simulink model "REALTIME_PART1_backwardEuler"  (R2020b)
settings: Solver=ode3  StartTime=0.0  StopTime=5  FixedStep=0.001  RelTol=1e-3
undefined symbols (not defined in the file or in its folder): ctrl, DiscIntNeverNeededParam, K_w, National_Instruments, PCI, sens, step_size, T, Tl
libraries: sldrtlib x2
settings Model: ExtModeTrigDuration=6000  Creator=gioel  LastModifiedBy=pavarinlau
settings DataIOCC: ReturnWorkspaceOutputs=off
settings RTWCC: Description=Simulink Desktop Real-Time  SystemTargetFile=sldrt.tlc  TemplateMakefile=sldrt.tmf  RTWCompilerOptimization=on
settings CodeAppCC: MaxIdLength=95
settings SimulinkDesktopRealTimeCC: TargetPreCompLibLocation=C:\Program Files\MATLAB\R2020b\toolbox\sldrt\lib\win64

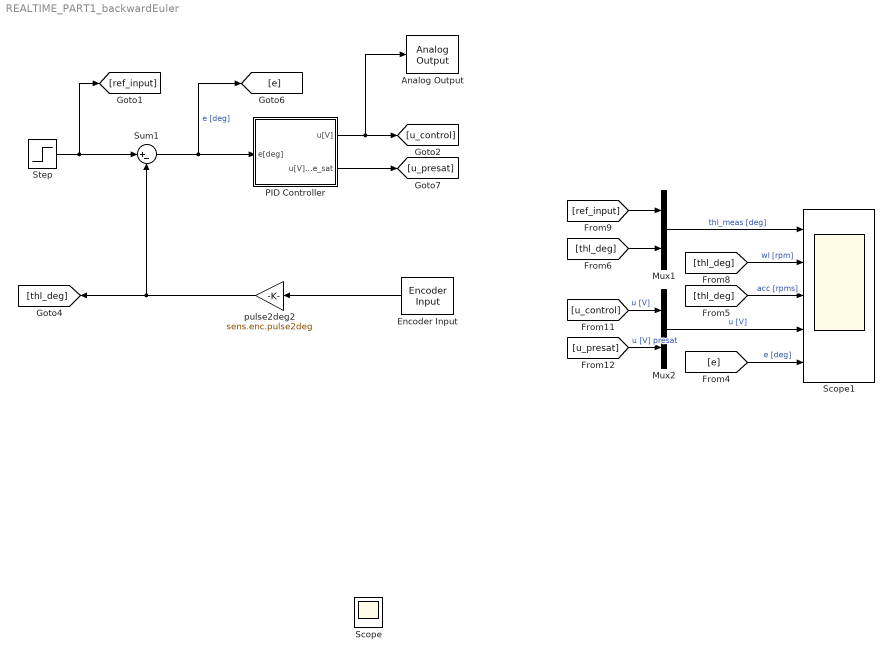
== system REALTIME_PART1_backwardEuler ==
  Analog Output : sldrtlib/Analog Output  SampleTime=-1  MaxMissedTicks=10  ShowMissedTicks=off  YieldWhenWaiting=off  DrvName=National_Instruments/PCI-6221  DrvAddress=4294967295  DrvOptions=[0 0 0 2 0]  Channels=1  RangeMode=1  VoltRange=1  InitialValue=0  FinalValue=0
      settings: AttributesFormatString=National Instruments\nPCI-6221 [auto]
  Encoder Input : sldrtlib/Encoder Input  SampleTime=T  MaxMissedTicks=10  ShowMissedTicks=off  YieldWhenWaiting=off  DrvName=National_Instruments/PCI-6221  DrvAddress=4294967295  DrvOptions=[0 0 0 2 0]  Channels=1  QuadMode=3  IndexPulse=1  InputFilter=Inf  DataType=1
      settings: AttributesFormatString=National Instruments\nPCI-6221 [auto]
  Mux1 : Mux  Inputs=2
  Mux2 : Mux  Inputs=2
  PID Controller : Subsystem
  Scope1 : Scope  NumInputPorts=5
  Step : Step  After=step_size  SampleTime=T
  Sum1 : Sum  Inputs=|+-
  pulse2deg2 : Gain  Gain=sens.enc.pulse2deg
  Scope : Scope
  wires:
  Sum1/1 -> [e], PID Controller/1(e[deg])  "e [deg]"
  Step/1 -> Sum1/1, [ref_input]
  PID Controller/1(u[V]) -> Analog Output/1, [u_control]
  Mux1/1 -> Scope1/1  "thl_meas [deg]"
  [thl_deg] -> Mux1/2
  [thl_deg] -> Scope1/3  "acc [rpms]"
  Mux2/1 -> Scope1/4  "u [V]"
  [thl_deg] -> Scope1/2  "wl [rpm]"
  [ref_input] -> Mux1/1
  pulse2deg2/1 -> Sum1/2, [thl_deg]
  [e] -> Scope1/5  "e [deg]"
  PID Controller/2(u[V] pre_sat) -> [u_presat]
  [u_control] -> Mux2/1  "u [V]"
  [u_presat] -> Mux2/2  "u [V] presat"
  Encoder Input/1 -> pulse2deg2/1

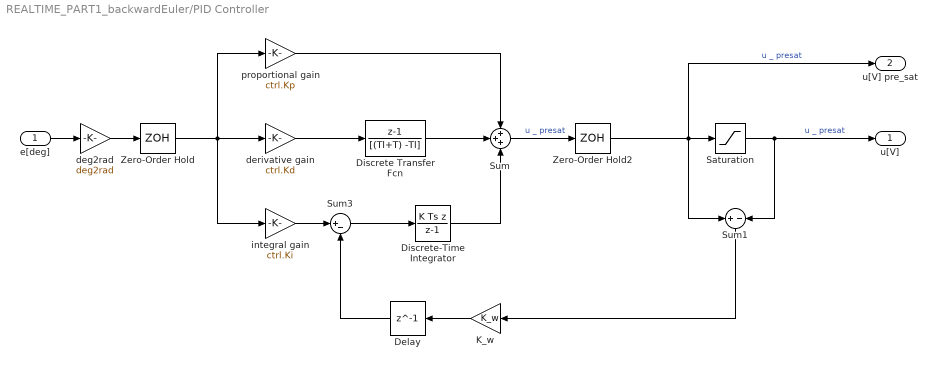
== system REALTIME_PART1_backwardEuler/PID Controller ==
  e[deg] : Inport
  Delay : Delay  DelayLength=1  InitialCondition=0  SampleTime=T
  Discrete Transfer Fcn : DiscreteTransferFcn  Numerator=[1 -1]  Denominator=[(Tl+T) -Tl]  SampleTime=T
  Discrete-Time Integrator : DiscreteIntegrator  IntegratorMethod=Integration: Backward Euler  SampleTime=T  ICPrevOutput=DiscIntNeverNeededParam  ICPrevScaledInput=DiscIntNeverNeededParam
  "K_w " : Gain  Gain=K_w
  Saturation : Saturate  UpperLimit=10  LowerLimit=-10
  Sum : Sum  Inputs=+++
  Sum1 : Sum  Inputs=+|-
  Sum3 : Sum  Inputs=|+-
  Zero-Order Hold : ZeroOrderHold  SampleTime=T
  Zero-Order Hold2 : ZeroOrderHold  SampleTime=T
  deg2rad : Gain  Gain=deg2rad
  derivative gain : Gain  Gain=ctrl.Kd
  integral gain : Gain  Gain=ctrl.Ki
  proportional gain : Gain  Gain=ctrl.Kp
  u[V] : Outport
  u[V] pre_sat : Outport  Port=2
  wires:
  proportional gain/1 -> Sum/1
  e[deg]/1 -> deg2rad/1
  deg2rad/1 -> Zero-Order Hold/1
  Zero-Order Hold/1 -> integral gain/1, derivative gain/1, proportional gain/1
  derivative gain/1 -> Discrete Transfer Fcn/1
  Discrete Transfer Fcn/1 -> Sum/2
  Discrete-Time Integrator/1 -> Sum/3
  Sum1/1 -> "K_w "/1
  integral gain/1 -> Sum3/1
  Sum3/1 -> Discrete-Time Integrator/1
  "K_w "/1 -> Delay/1
  Sum/1 -> Zero-Order Hold2/1  "u _ presat"
  Saturation/1 -> u[V]/1, Sum1/2  "u _ presat"
  Zero-Order Hold2/1 -> u[V] pre_sat/1, Sum1/1, Saturation/1  "u _ presat"
  Delay/1 -> Sum3/2
